simulink model "frontModel"  (R2020b)
settings: Solver=VariableStepAuto  StartTime=0.0  StopTime=10.0  RelTol=1e-3
model workspace: external: MATLAB File C:\Code\KillerWhaleSim\KillerWhaleSim\FrontParams.m (data not in the file)
undefined symbols (not defined in the file or in its folder): frontParams, X, Y, Z
libraries: sm_lib x1214, nesl_utility x1
(part 1 of 19)
settings Model: Creator=roadrunner  LastModifiedBy=roadrunner

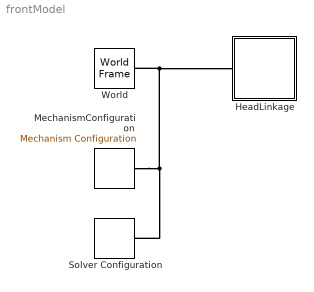
== system frontModel ==
  HeadLinkage : Subsystem
  MechanismConfiguration : sm_lib/Utilities/Mechanism Configuration  UniformGravity=Constant  GravityVector=[0 -9.80665 0]  GravityVectorUnits=m/s^2  GravityUnits=m/s^2  LinearizationDelta=0.001  JointModeTransitionNonlinearIterations=2
  Solver Configuration : nesl_utility/Solver Configuration  PhysicalDomain=network_engine_domain  SubClassName=solver  LeftPortType=input  RightPortType=generic  Tones=[]  Harmonics=[]  SimulateNoise=off  Profile=off  UseLocalSampling=off  EnableSwitchedLinearOptims=on  FrequencyDomain=off  UseCCode=off  RelTol=0.001  AbsTol=1e-06  MinStep=1e-09  ToWorkspace=off  RevertToSquareIcSolve=off  NumHomotopyIterations=100  PhasorMode=off  PhasorModeNumHarmonics=1  DoDC=off  ResidualTolerance=1e-09  UseLocalSolver=off  LocalSolverChoice=NE_BACKWARD_EULER_ADVANCER  LocalSolverSampleTime=0.001  DoFixedCost=off  MaxNonlinIter=3  MaxModeIter=2  ComputeImpulses=off  ImpulseIterations=2  LinearAlgebra=auto  EquationFormulation=NE_TIME_EF  DelaysMemoryBudget=1024  AutomaticFiltering=on  FilteringTimeConstant=0.001  PartitionStorageMethod=AS_NEEDED  PartitionMemoryBudget=1024  PartitionMethod=ROBUST
  World : sm_lib/Frames and Transforms/World Frame
  connections:
  World/RConn1 -- MechanismConfiguration/RConn1 -- Solver Configuration/RConn1 -- HeadLinkage/LConn1

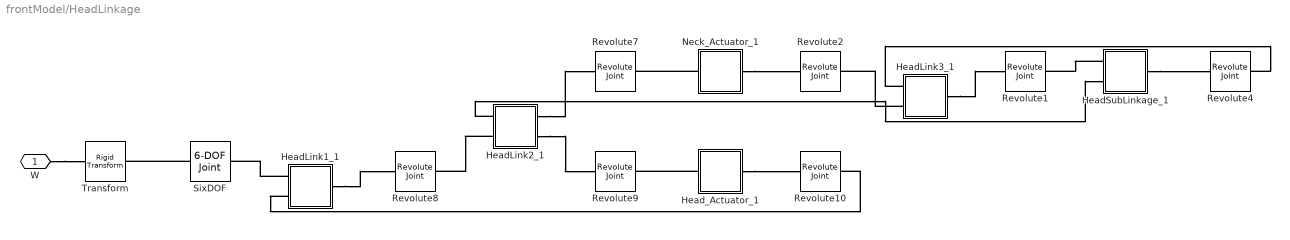
== system frontModel/HeadLinkage ==
  HeadLink1_1 : Subsystem
  HeadLink2_1 : Subsystem
  HeadLink3_1 : Subsystem
  HeadSubLinkage_1 : Subsystem
  Head_Actuator_1 : Subsystem
  Neck_Actuator_1 : Subsystem
  Revolute1 : sm_lib/Joints/Revolute Joint  JointMode=Normal  SenseConstraintForce=off  SenseConstraintForceX=off  SenseConstraintForceY=off  SenseConstraintForceZ=off  SenseConstraintTorque=off  SenseConstraintTorqueX=off  SenseConstraintTorqueY=off  SenseConstraintTorqueZ=off  SenseTotalForce=off  SenseTotalForceX=off  SenseTotalForceY=off  SenseTotalForceZ=off  SenseTotalTorque=off  SenseTotalTorqueX=off  SenseTotalTorqueY=off  SenseTotalTorqueZ=off  CompositeWrenchDir=FollowerOnBase  CompositeWrenchFrame=BaseFrame  EquilibriumPosition=0  EquilibriumPositionUnits=deg  SpringStiffness=0  SpringStiffnessUnits=N*m/deg  DampingCoefficient=0  DampingCoefficientUnits=N*m/(deg/s)  TorqueActuationMode=NoTorque  MotionActuationMode=ComputedMotion  SensePosition=off  SenseVelocity=off  SenseAcceleration=off  SenseTorqueForce=off  SenseLowerLimitTorqueForce=off  SenseUpperLimitTorqueForce=off  LowerLimitSpecify=off  LowerLimitBound=-90  LowerLimitBoundUnits=deg  LowerLimitStiffness=1e4  LowerLimitStiffnessUnits=N*m/deg  LowerLimitDamping=10  LowerLimitDampingUnits=N*m/(deg/s)  LowerLimitTransitionRegionWidth=0.1  LowerLimitTransitionRegionWidthUnits=deg  UpperLimitSpecify=off  UpperLimitBound=90  UpperLimitBoundUnits=deg  UpperLimitStiffness=1e4  UpperLimitStiffnessUnits=N*m/deg  UpperLimitDamping=10  UpperLimitDampingUnits=N*m/(deg/s)  UpperLimitTransitionRegionWidth=0.1  UpperLimitTransitionRegionWidthUnits=deg  PositionTargetSpecify=on  PositionTargetPriority=Low  PositionTargetValue=frontParams.RevoluteJoint(8).Rz.Pos  PositionTargetValueUnits=deg  VelocityTargetSpecify=off  VelocityTargetPriority=High  VelocityTargetValue=0  VelocityTargetValueUnits=deg/s
  Revolute10 : sm_lib/Joints/Revolute Joint  JointMode=Normal  SenseConstraintForce=off  SenseConstraintForceX=off  SenseConstraintForceY=off  SenseConstraintForceZ=off  SenseConstraintTorque=off  SenseConstraintTorqueX=off  SenseConstraintTorqueY=off  SenseConstraintTorqueZ=off  SenseTotalForce=off  SenseTotalForceX=off  SenseTotalForceY=off  SenseTotalForceZ=off  SenseTotalTorque=off  SenseTotalTorqueX=off  SenseTotalTorqueY=off  SenseTotalTorqueZ=off  CompositeWrenchDir=FollowerOnBase  CompositeWrenchFrame=BaseFrame  EquilibriumPosition=0  EquilibriumPositionUnits=deg  SpringStiffness=0  SpringStiffnessUnits=N*m/deg  DampingCoefficient=0  DampingCoefficientUnits=N*m/(deg/s)  TorqueActuationMode=NoTorque  MotionActuationMode=ComputedMotion  SensePosition=off  SenseVelocity=off  SenseAcceleration=off  SenseTorqueForce=off  SenseLowerLimitTorqueForce=off  SenseUpperLimitTorqueForce=off  LowerLimitSpecify=off  LowerLimitBound=-90  LowerLimitBoundUnits=deg  LowerLimitStiffness=1e4  LowerLimitStiffnessUnits=N*m/deg  LowerLimitDamping=10  LowerLimitDampingUnits=N*m/(deg/s)  LowerLimitTransitionRegionWidth=0.1  LowerLimitTransitionRegionWidthUnits=deg  UpperLimitSpecify=off  UpperLimitBound=90  UpperLimitBoundUnits=deg  UpperLimitStiffness=1e4  UpperLimitStiffnessUnits=N*m/deg  UpperLimitDamping=10  UpperLimitDampingUnits=N*m/(deg/s)  UpperLimitTransitionRegionWidth=0.1  UpperLimitTransitionRegionWidthUnits=deg  PositionTargetSpecify=on  PositionTargetPriority=Low  PositionTargetValue=frontParams.RevoluteJoint(5).Rz.Pos  PositionTargetValueUnits=deg  VelocityTargetSpecify=off  VelocityTargetPriority=High  VelocityTargetValue=0  VelocityTargetValueUnits=deg/s
  Revolute2 : sm_lib/Joints/Revolute Joint  JointMode=Normal  SenseConstraintForce=off  SenseConstraintForceX=off  SenseConstraintForceY=off  SenseConstraintForceZ=off  SenseConstraintTorque=off  SenseConstraintTorqueX=off  SenseConstraintTorqueY=off  SenseConstraintTorqueZ=off  SenseTotalForce=off  SenseTotalForceX=off  SenseTotalForceY=off  SenseTotalForceZ=off  SenseTotalTorque=off  SenseTotalTorqueX=off  SenseTotalTorqueY=off  SenseTotalTorqueZ=off  CompositeWrenchDir=FollowerOnBase  CompositeWrenchFrame=BaseFrame  EquilibriumPosition=0  EquilibriumPositionUnits=deg  SpringStiffness=0  SpringStiffnessUnits=N*m/deg  DampingCoefficient=0  DampingCoefficientUnits=N*m/(deg/s)  TorqueActuationMode=NoTorque  MotionActuationMode=ComputedMotion  SensePosition=off  SenseVelocity=off  SenseAcceleration=off  SenseTorqueForce=off  SenseLowerLimitTorqueForce=off  SenseUpperLimitTorqueForce=off  LowerLimitSpecify=off  LowerLimitBound=-90  LowerLimitBoundUnits=deg  LowerLimitStiffness=1e4  LowerLimitStiffnessUnits=N*m/deg  LowerLimitDamping=10  LowerLimitDampingUnits=N*m/(deg/s)  LowerLimitTransitionRegionWidth=0.1  LowerLimitTransitionRegionWidthUnits=deg  UpperLimitSpecify=off  UpperLimitBound=90  UpperLimitBoundUnits=deg  UpperLimitStiffness=1e4  UpperLimitStiffnessUnits=N*m/deg  UpperLimitDamping=10  UpperLimitDampingUnits=N*m/(deg/s)  UpperLimitTransitionRegionWidth=0.1  UpperLimitTransitionRegionWidthUnits=deg  PositionTargetSpecify=off  PositionTargetPriority=High  PositionTargetValue=0  PositionTargetValueUnits=deg  VelocityTargetSpecify=off  VelocityTargetPriority=High  VelocityTargetValue=0  VelocityTargetValueUnits=deg/s
  Revolute4 : sm_lib/Joints/Revolute Joint  JointMode=Normal  SenseConstraintForce=off  SenseConstraintForceX=off  SenseConstraintForceY=off  SenseConstraintForceZ=off  SenseConstraintTorque=off  SenseConstraintTorqueX=off  SenseConstraintTorqueY=off  SenseConstraintTorqueZ=off  SenseTotalForce=off  SenseTotalForceX=off  SenseTotalForceY=off  SenseTotalForceZ=off  SenseTotalTorque=off  SenseTotalTorqueX=off  SenseTotalTorqueY=off  SenseTotalTorqueZ=off  CompositeWrenchDir=FollowerOnBase  CompositeWrenchFrame=BaseFrame  EquilibriumPosition=0  EquilibriumPositionUnits=deg  SpringStiffness=0  SpringStiffnessUnits=N*m/deg  DampingCoefficient=0  DampingCoefficientUnits=N*m/(deg/s)  TorqueActuationMode=NoTorque  MotionActuationMode=ComputedMotion  SensePosition=off  SenseVelocity=off  SenseAcceleration=off  SenseTorqueForce=off  SenseLowerLimitTorqueForce=off  SenseUpperLimitTorqueForce=off  LowerLimitSpecify=off  LowerLimitBound=-90  LowerLimitBoundUnits=deg  LowerLimitStiffness=1e4  LowerLimitStiffnessUnits=N*m/deg  LowerLimitDamping=10  LowerLimitDampingUnits=N*m/(deg/s)  LowerLimitTransitionRegionWidth=0.1  LowerLimitTransitionRegionWidthUnits=deg  UpperLimitSpecify=off  UpperLimitBound=90  UpperLimitBoundUnits=deg  UpperLimitStiffness=1e4  UpperLimitStiffnessUnits=N*m/deg  UpperLimitDamping=10  UpperLimitDampingUnits=N*m/(deg/s)  UpperLimitTransitionRegionWidth=0.1  UpperLimitTransitionRegionWidthUnits=deg  PositionTargetSpecify=on  PositionTargetPriority=Low  PositionTargetValue=frontParams.RevoluteJoint(7).Rz.Pos  PositionTargetValueUnits=deg  VelocityTargetSpecify=off  VelocityTargetPriority=High  VelocityTargetValue=0  VelocityTargetValueUnits=deg/s
  Revolute7 : sm_lib/Joints/Revolute Joint  JointMode=Normal  SenseConstraintForce=off  SenseConstraintForceX=off  SenseConstraintForceY=off  SenseConstraintForceZ=off  SenseConstraintTorque=off  SenseConstraintTorqueX=off  SenseConstraintTorqueY=off  SenseConstraintTorqueZ=off  SenseTotalForce=off  SenseTotalForceX=off  SenseTotalForceY=off  SenseTotalForceZ=off  SenseTotalTorque=off  SenseTotalTorqueX=off  SenseTotalTorqueY=off  SenseTotalTorqueZ=off  CompositeWrenchDir=FollowerOnBase  CompositeWrenchFrame=BaseFrame  EquilibriumPosition=0  EquilibriumPositionUnits=deg  SpringStiffness=0  SpringStiffnessUnits=N*m/deg  DampingCoefficient=0  DampingCoefficientUnits=N*m/(deg/s)  TorqueActuationMode=NoTorque  MotionActuationMode=ComputedMotion  SensePosition=off  SenseVelocity=off  SenseAcceleration=off  SenseTorqueForce=off  SenseLowerLimitTorqueForce=off  SenseUpperLimitTorqueForce=off  LowerLimitSpecify=off  LowerLimitBound=-90  LowerLimitBoundUnits=deg  LowerLimitStiffness=1e4  LowerLimitStiffnessUnits=N*m/deg  LowerLimitDamping=10  LowerLimitDampingUnits=N*m/(deg/s)  LowerLimitTransitionRegionWidth=0.1  LowerLimitTransitionRegionWidthUnits=deg  UpperLimitSpecify=off  UpperLimitBound=90  UpperLimitBoundUnits=deg  UpperLimitStiffness=1e4  UpperLimitStiffnessUnits=N*m/deg  UpperLimitDamping=10  UpperLimitDampingUnits=N*m/(deg/s)  UpperLimitTransitionRegionWidth=0.1  UpperLimitTransitionRegionWidthUnits=deg  PositionTargetSpecify=on  PositionTargetPriority=Low  PositionTargetValue=frontParams.RevoluteJoint(9).Rz.Pos  PositionTargetValueUnits=deg  VelocityTargetSpecify=off  VelocityTargetPriority=High  VelocityTargetValue=0  VelocityTargetValueUnits=deg/s
  Revolute8 : sm_lib/Joints/Revolute Joint  JointMode=Normal  SenseConstraintForce=off  SenseConstraintForceX=off  SenseConstraintForceY=off  SenseConstraintForceZ=off  SenseConstraintTorque=off  SenseConstraintTorqueX=off  SenseConstraintTorqueY=off  SenseConstraintTorqueZ=off  SenseTotalForce=off  SenseTotalForceX=off  SenseTotalForceY=off  SenseTotalForceZ=off  SenseTotalTorque=off  SenseTotalTorqueX=off  SenseTotalTorqueY=off  SenseTotalTorqueZ=off  CompositeWrenchDir=FollowerOnBase  CompositeWrenchFrame=BaseFrame  EquilibriumPosition=0  EquilibriumPositionUnits=deg  SpringStiffness=0  SpringStiffnessUnits=N*m/deg  DampingCoefficient=0  DampingCoefficientUnits=N*m/(deg/s)  TorqueActuationMode=NoTorque  MotionActuationMode=ComputedMotion  SensePosition=off  SenseVelocity=off  SenseAcceleration=off  SenseTorqueForce=off  SenseLowerLimitTorqueForce=off  SenseUpperLimitTorqueForce=off  LowerLimitSpecify=off  LowerLimitBound=-90  LowerLimitBoundUnits=deg  LowerLimitStiffness=1e4  LowerLimitStiffnessUnits=N*m/deg  LowerLimitDamping=10  LowerLimitDampingUnits=N*m/(deg/s)  LowerLimitTransitionRegionWidth=0.1  LowerLimitTransitionRegionWidthUnits=deg  UpperLimitSpecify=off  UpperLimitBound=90  UpperLimitBoundUnits=deg  UpperLimitStiffness=1e4  UpperLimitStiffnessUnits=N*m/deg  UpperLimitDamping=10  UpperLimitDampingUnits=N*m/(deg/s)  UpperLimitTransitionRegionWidth=0.1  UpperLimitTransitionRegionWidthUnits=deg  PositionTargetSpecify=on  PositionTargetPriority=Low  PositionTargetValue=frontParams.RevoluteJoint(6).Rz.Pos  PositionTargetValueUnits=deg  VelocityTargetSpecify=off  VelocityTargetPriority=High  VelocityTargetValue=0  VelocityTargetValueUnits=deg/s
  Revolute9 : sm_lib/Joints/Revolute Joint  JointMode=Normal  SenseConstraintForce=off  SenseConstraintForceX=off  SenseConstraintForceY=off  SenseConstraintForceZ=off  SenseConstraintTorque=off  SenseConstraintTorqueX=off  SenseConstraintTorqueY=off  SenseConstraintTorqueZ=off  SenseTotalForce=off  SenseTotalForceX=off  SenseTotalForceY=off  SenseTotalForceZ=off  SenseTotalTorque=off  SenseTotalTorqueX=off  SenseTotalTorqueY=off  SenseTotalTorqueZ=off  CompositeWrenchDir=FollowerOnBase  CompositeWrenchFrame=BaseFrame  EquilibriumPosition=0  EquilibriumPositionUnits=deg  SpringStiffness=0  SpringStiffnessUnits=N*m/deg  DampingCoefficient=0  DampingCoefficientUnits=N*m/(deg/s)  TorqueActuationMode=NoTorque  MotionActuationMode=ComputedMotion  SensePosition=off  SenseVelocity=off  SenseAcceleration=off  SenseTorqueForce=off  SenseLowerLimitTorqueForce=off  SenseUpperLimitTorqueForce=off  LowerLimitSpecify=off  LowerLimitBound=-90  LowerLimitBoundUnits=deg  LowerLimitStiffness=1e4  LowerLimitStiffnessUnits=N*m/deg  LowerLimitDamping=10  LowerLimitDampingUnits=N*m/(deg/s)  LowerLimitTransitionRegionWidth=0.1  LowerLimitTransitionRegionWidthUnits=deg  UpperLimitSpecify=off  UpperLimitBound=90  UpperLimitBoundUnits=deg  UpperLimitStiffness=1e4  UpperLimitStiffnessUnits=N*m/deg  UpperLimitDamping=10  UpperLimitDampingUnits=N*m/(deg/s)  UpperLimitTransitionRegionWidth=0.1  UpperLimitTransitionRegionWidthUnits=deg  PositionTargetSpecify=off  PositionTargetPriority=High  PositionTargetValue=0  PositionTargetValueUnits=deg  VelocityTargetSpecify=off  VelocityTargetPriority=High  VelocityTargetValue=0  VelocityTargetValueUnits=deg/s
  SixDOF : sm_lib/Joints/6-DOF Joint  JointMode=Normal  SenseConstraintForce=off  SenseConstraintForceX=off  SenseConstraintForceY=off  SenseConstraintForceZ=off  SenseConstraintTorque=off  SenseConstraintTorqueX=off  SenseConstraintTorqueY=off  SenseConstraintTorqueZ=off  SenseTotalForce=off  SenseTotalForceX=off  SenseTotalForceY=off  SenseTotalForceZ=off  SenseTotalTorque=off  SenseTotalTorqueX=off  SenseTotalTorqueY=off  SenseTotalTorqueZ=off  CompositeWrenchDir=FollowerOnBase  CompositeWrenchFrame=BaseFrame  PxEquilibriumPosition=0  PxEquilibriumPositionUnits=m  PxSpringStiffness=0  PxSpringStiffnessUnits=N/m  PxDampingCoefficient=0  PxDampingCoefficientUnits=N/(m/s)  PxTorqueActuationMode=NoTorque  PxMotionActuationMode=ComputedMotion  PxSensePosition=off  PxSenseVelocity=off  PxSenseAcceleration=off  PxSenseTorqueForce=off  PxSenseLowerLimitTorqueForce=off  PxSenseUpperLimitTorqueForce=off  PxLowerLimitSpecify=off  PxLowerLimitBound=-1  PxLowerLimitBoundUnits=m  PxLowerLimitStiffness=1e6  PxLowerLimitStiffnessUnits=N/m  PxLowerLimitDamping=1e3  PxLowerLimitDampingUnits=N/(m/s)  PxLowerLimitTransitionRegionWidth=1e-4  PxLowerLimitTransitionRegionWidthUnits=m  PxUpperLimitSpecify=off  PxUpperLimitBound=1  PxUpperLimitBoundUnits=m  PxUpperLimitStiffness=1e6  PxUpperLimitStiffnessUnits=N/m  PxUpperLimitDamping=1e3  PxUpperLimitDampingUnits=N/(m/s)  PxUpperLimitTransitionRegionWidth=1e-4  PxUpperLimitTransitionRegionWidthUnits=m  PxPositionTargetSpecify=off  PxPositionTargetPriority=High  PxPositionTargetValue=0  PxPositionTargetValueUnits=m  PxVelocityTargetSpecify=off  PxVelocityTargetPriority=High  PxVelocityTargetValue=0  PxVelocityTargetValueUnits=m/s  PyEquilibriumPosition=0  PyEquilibriumPositionUnits=m  PySpringStiffness=0  PySpringStiffnessUnits=N/m  PyDampingCoefficient=0  PyDampingCoefficientUnits=N/(m/s)  PyTorqueActuationMode=NoTorque  PyMotionActuationMode=ComputedMotion  PySensePosition=off  PySenseVelocity=off  PySenseAcceleration=off  PySenseTorqueForce=off  PySenseLowerLimitTorqueForce=off  PySenseUpperLimitTorqueForce=off  PyLowerLimitSpecify=off  PyLowerLimitBound=-1  PyLowerLimitBoundUnits=m  PyLowerLimitStiffness=1e6  PyLowerLimitStiffnessUnits=N/m  PyLowerLimitDamping=1e3  PyLowerLimitDampingUnits=N/(m/s)  PyLowerLimitTransitionRegionWidth=1e-4  PyLowerLimitTransitionRegionWidthUnits=m  PyUpperLimitSpecify=off  PyUpperLimitBound=1  PyUpperLimitBoundUnits=m  PyUpperLimitStiffness=1e6  PyUpperLimitStiffnessUnits=N/m  PyUpperLimitDamping=1e3  PyUpperLimitDampingUnits=N/(m/s)  PyUpperLimitTransitionRegionWidth=1e-4  PyUpperLimitTransitionRegionWidthUnits=m  PyPositionTargetSpecify=off  PyPositionTargetPriority=High  PyPositionTargetValue=0  PyPositionTargetValueUnits=m  PyVelocityTargetSpecify=off  PyVelocityTargetPriority=High  PyVelocityTargetValue=0  PyVelocityTargetValueUnits=m/s  PzEquilibriumPosition=0  PzEquilibriumPositionUnits=m  PzSpringStiffness=0  PzSpringStiffnessUnits=N/m  PzDampingCoefficient=0  PzDampingCoefficientUnits=N/(m/s)  PzTorqueActuationMode=NoTorque  PzMotionActuationMode=ComputedMotion  PzSensePosition=off  PzSenseVelocity=off  PzSenseAcceleration=off  PzSenseTorqueForce=off  PzSenseLowerLimitTorqueForce=off  PzSenseUpperLimitTorqueForce=off  PzLowerLimitSpecify=off  PzLowerLimitBound=-1  PzLowerLimitBoundUnits=m  PzLowerLimitStiffness=1e6  PzLowerLimitStiffnessUnits=N/m  PzLowerLimitDamping=1e3  PzLowerLimitDampingUnits=N/(m/s)  PzLowerLimitTransitionRegionWidth=1e-4  PzLowerLimitTransitionRegionWidthUnits=m  PzUpperLimitSpecify=off  PzUpperLimitBound=1  PzUpperLimitBoundUnits=m  PzUpperLimitStiffness=1e6  PzUpperLimitStiffnessUnits=N/m  PzUpperLimitDamping=1e3  PzUpperLimitDampingUnits=N/(m/s)  PzUpperLimitTransitionRegionWidth=1e-4  PzUpperLimitTransitionRegionWidthUnits=m  PzPositionTargetSpecify=off  PzPositionTargetPriority=High  PzPositionTargetValue=0  PzPositionTargetValueUnits=m  PzVelocityTargetSpecify=off  PzVelocityTargetPriority=High  PzVelocityTargetValue=0  PzVelocityTargetValueUnits=m/s  SphDefPosRotationMethod=None  SphDefPosRotationAngleUnits=deg  SphDefPosRotationStandardAxis=+Z  SphDefPosRotationAngle=0.0  SphDefPosRotationArbitraryAxis=[0 0 1]  SphDefPosFollAlignAxisA=+X  SphDefPosBaseAlignAxisA=+Y  SphDefPosFollAlignAxisB=+Y  SphDefPosBaseAlignAxisB=+Z  SphDefPosRotationSequenceAxes=FollowerAxes  SphDefPosRotationSequence=XYX  SphDefPosRotationSequenceAngles=[0 0 0]  SphDefPosRotationSequenceAnglesUnits=deg  SphDefPosRotationMatrix=[1 0 0; 0 1 0; 0 0 1]  SphEqPosRotationMethod=None  SphEqPosRotationAngleUnits=deg  SphEqPosRotationStandardAxis=+Z  SphEqPosRotationAngle=0.0  SphEqPosRotationArbitraryAxis=[0 0 1]  SphEqPosFollAlignAxisA=+X  SphEqPosBaseAlignAxisA=+Y  SphEqPosFollAlignAxisB=+Y  SphEqPosBaseAlignAxisB=+Z  SphEqPosRotationSequenceAxes=FollowerAxes  SphEqPosRotationSequence=XYX  SphEqPosRotationSequenceAngles=[0 0 0]  SphEqPosRotationSequenceAnglesUnits=deg  SphEqPosRotationMatrix=[1 0 0; 0 1 0; 0 0 1]  SphSpringStiffness=0  SphSpringStiffnessUnits=N*m/deg  SphDampingCoefficient=0  SphDampingCoefficientUnits=N*m/(deg/s)  SphActuateTorqueX=off  SphActuateTorqueY=off  SphActuateTorqueZ=off  SphActuateTorque=off  SphTorqueActuationMode=NoTorque  SphMotionActuationMode=ComputedMotion  SphActuationFrame=BaseFrame  SphSensePosition=off  SphSenseVelocityX=off  SphSenseVelocityY=off  SphSenseVelocityZ=off  SphSenseVelocity=off  SphSenseAccelerationX=off  SphSenseAccelerationY=off  SphSenseAccelerationZ=off  SphSenseAcceleration=off  SphSenseTorqueX=off  SphSenseTorqueY=off  SphSenseTorqueZ=off  SphSenseTorqueForce=off  SphSenseLowerLimitTorqueMag=off  SphSenseUpperLimitTorqueMag=off  SphSensingFrame=FollowerFrame  SphLowerLimitSpecify=off  SphLowerLimitBound=15  SphLowerLimitBoundUnits=deg  SphLowerLimitStiffness=1e4  SphLowerLimitStiffnessUnits=N*m/deg  SphLowerLimitDamping=10  SphLowerLimitDampingUnits=N*m/(deg/s)  SphLowerLimitTransitionRegionWidth=0.1  SphLowerLimitTransitionRegionWidthUnits=deg  SphUpperLimitSpecify=off  SphUpperLimitBound=45  SphUpperLimitBoundUnits=deg  SphUpperLimitStiffness=1e4  SphUpperLimitStiffnessUnits=N*m/deg  SphUpperLimitDamping=10  SphUpperLimitDampingUnits=N*m/(deg/s)  SphUpperLimitTransitionRegionWidth=0.1  SphUpperLimitTransitionRegionWidthUnits=deg  SphPositionTargetRotationMethod=None  SphPositionTargetRotationAngleUnits=deg  SphPositionTargetRotationStandardAxis=+Z  SphPositionTargetRotationAngle=0.0  SphPositionTargetRotationArbitraryAxis=[0 0 1]  SphPositionTargetFollAlignAxisA=+X  SphPositionTargetBaseAlignAxisA=+Y  SphPositionTargetFollAlignAxisB=+Y  SphPositionTargetBaseAlignAxisB=+Z  SphPositionTargetRotationSequenceAxes=FollowerAxes  SphPositionTargetRotationSequence=XYX  SphPositionTargetRotationSequenceAngles=[0 0 0]  SphPositionTargetRotationSequenceAnglesUnits=deg  SphPositionTargetRotationMatrix=[1 0 0; 0 1 0; 0 0 1]  SphPositionTargetSpecify=off  SphPositionTargetPriority=High  SphVelocityTargetValue=[0 0 0]  SphVelocityTargetValueUnits=deg/s  SphVelocityTargetSpecify=off  SphVelocityTargetPriority=High  SphVelocityTargetInFollowerFrame=on
  Transform : sm_lib/Frames and Transforms/Rigid Transform  TranslationMethod=Cartesian  TranslationStandardOffset=0  TranslationLengthUnit=in  TranslationStandardAxis=+Z  TranslationCartesianOffset=frontParams.RigidTransform(423).translation  TranslationROffset=0  TranslationROffsetUnits=m  TranslationZOffset=0  TranslationZOffsetUnits=m  TranslationThetaOffset=0  TranslationThetaOffsetUnits=deg  RotationMethod=ArbitraryAxis  RotationAngleUnits=rad  RotationStandardAxis=+Z  RotationAngle=frontParams.RigidTransform(423).angle  RotationArbitraryAxis=frontParams.RigidTransform(423).axis  FollAlignAxisA=+X  BaseAlignAxisA=+Y  FollAlignAxisB=+Y  BaseAlignAxisB=+Z  RotationSequenceAxes=FollowerAxes  RotationSequence=XYX  RotationSequenceAngles=[0 0 0]  RotationSequenceAnglesUnits=deg  RotationMatrix=[1 0 0; 0 1 0; 0 0 1]
  W : PMIOPort  Side=Left
  connections:
  HeadSubLinkage_1/LConn1 -- Revolute1/RConn1
  HeadLink2_1/RConn2 -- Revolute9/LConn1
  Head_Actuator_1/RConn1 -- Revolute10/LConn1
  Neck_Actuator_1/LConn1 -- Revolute7/RConn1
  HeadLink2_1/LConn2 -- Revolute8/RConn1
  HeadLink1_1/RConn1 -- Revolute8/LConn1
  HeadLink3_1/LConn1 -- Revolute4/RConn1
  HeadLink1_1/LConn1 -- SixDOF/RConn1
  SixDOF/LConn1 -- Transform/RConn1
  HeadLink1_1/LConn2 -- Revolute10/RConn1
  HeadSubLinkage_1/RConn1 -- Revolute4/LConn1
  HeadLink2_1/LConn1 -- HeadSubLinkage_1/LConn2
  Head_Actuator_1/LConn1 -- Revolute9/RConn1
  Neck_Actuator_1/RConn1 -- Revolute2/LConn1
  HeadLink3_1/RConn1 -- Revolute1/LConn1
  HeadLink3_1/LConn2 -- Revolute2/RConn1
  HeadLink2_1/RConn1 -- Revolute7/LConn1
  W/RConn1 -- Transform/LConn1

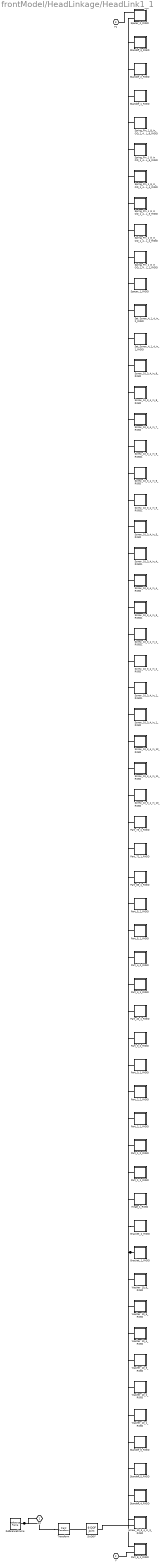
== system frontModel/HeadLinkage/HeadLink1_1 ==
  Bracket_1_RIGID : Subsystem
  Bracket_2_RIGID : Subsystem
  Hinge_1_RIGID : Subsystem
  Part_1_1_RIGID : Subsystem
  Part_1_2_RIGID : Subsystem
  Part_2_1_RIGID : Subsystem
  Part_2_2_RIGID : Subsystem
  Part_3_1_RIGID : Subsystem
  Part_3_2_RIGID : Subsystem
  Part_40_1_RIGID : Subsystem
  Part_4_1_RIGID : Subsystem
  Part_4_2_RIGID : Subsystem
  Part_5_1_RIGID : Subsystem
  Part_5_2_RIGID : Subsystem
  Part_65_1_RIGID : Subsystem
  Part_6_1_RIGID : Subsystem
  Part_72_1_RIGID : Subsystem
  Part_73_1_RIGID : Subsystem
  ReferenceFrame : sm_lib/Frames and Transforms/Reference Frame
  Screw_10_3_4_in_10_RIGID : Subsystem
  Screw_10_3_4_in_11_RIGID : Subsystem
  Screw_10_3_4_in_12_RIGID : Subsystem
  Screw_10_3_4_in_1_RIGID : Subsystem
  Screw_10_3_4_in_1_RIGID1 : Subsystem
  Screw_10_3_4_in_2_RIGID : Subsystem
  Screw_10_3_4_in_2_RIGID1 : Subsystem
  Screw_10_3_4_in_3_RIGID : Subsystem
  Screw_10_3_4_in_3_RIGID1 : Subsystem
  Screw_10_3_4_in_4_RIGID : Subsystem
  Screw_10_3_4_in_4_RIGID1 : Subsystem
  Screw_10_3_4_in_5_RIGID : Subsystem
  Screw_10_3_4_in_5_RIGID1 : Subsystem
  Screw_10_3_4_in_6_RIGID : Subsystem
  Screw_10_3_4_in_6_RIGID1 : Subsystem
  Screw_10_3_4_in_7_RIGID : Subsystem
  Screw_10_3_4_in_8_RIGID : Subsystem
  Screw_10_3_4_in_9_RIGID : Subsystem
  Set_Screw_4_1_4_in_1_RIGID : Subsystem
  Set_Screw_4_1_4_in_2_RIGID : Subsystem
  SixDOF : sm_lib/Joints/6-DOF Joint  JointMode=Normal  SenseConstraintForce=off  SenseConstraintForceX=off  SenseConstraintForceY=off  SenseConstraintForceZ=off  SenseConstraintTorque=off  SenseConstraintTorqueX=off  SenseConstraintTorqueY=off  SenseConstraintTorqueZ=off  SenseTotalForce=off  SenseTotalForceX=off  SenseTotalForceY=off  SenseTotalForceZ=off  SenseTotalTorque=off  SenseTotalTorqueX=off  SenseTotalTorqueY=off  SenseTotalTorqueZ=off  CompositeWrenchDir=FollowerOnBase  CompositeWrenchFrame=BaseFrame  PxEquilibriumPosition=0  PxEquilibriumPositionUnits=m  PxSpringStiffness=0  PxSpringStiffnessUnits=N/m  PxDampingCoefficient=0  PxDampingCoefficientUnits=N/(m/s)  PxTorqueActuationMode=NoTorque  PxMotionActuationMode=ComputedMotion  PxSensePosition=off  PxSenseVelocity=off  PxSenseAcceleration=off  PxSenseTorqueForce=off  PxSenseLowerLimitTorqueForce=off  PxSenseUpperLimitTorqueForce=off  PxLowerLimitSpecify=off  PxLowerLimitBound=-1  PxLowerLimitBoundUnits=m  PxLowerLimitStiffness=1e6  PxLowerLimitStiffnessUnits=N/m  PxLowerLimitDamping=1e3  PxLowerLimitDampingUnits=N/(m/s)  PxLowerLimitTransitionRegionWidth=1e-4  PxLowerLimitTransitionRegionWidthUnits=m  PxUpperLimitSpecify=off  PxUpperLimitBound=1  PxUpperLimitBoundUnits=m  PxUpperLimitStiffness=1e6  PxUpperLimitStiffnessUnits=N/m  PxUpperLimitDamping=1e3  PxUpperLimitDampingUnits=N/(m/s)  PxUpperLimitTransitionRegionWidth=1e-4  PxUpperLimitTransitionRegionWidthUnits=m  PxPositionTargetSpecify=off  PxPositionTargetPriority=High  PxPositionTargetValue=0  PxPositionTargetValueUnits=m  PxVelocityTargetSpecify=off  PxVelocityTargetPriority=High  PxVelocityTargetValue=0  PxVelocityTargetValueUnits=m/s  PyEquilibriumPosition=0  PyEquilibriumPositionUnits=m  PySpringStiffness=0  PySpringStiffnessUnits=N/m  PyDampingCoefficient=0  PyDampingCoefficientUnits=N/(m/s)  PyTorqueActuationMode=NoTorque  PyMotionActuationMode=ComputedMotion  PySensePosition=off  PySenseVelocity=off  PySenseAcceleration=off  PySenseTorqueForce=off  PySenseLowerLimitTorqueForce=off  PySenseUpperLimitTorqueForce=off  PyLowerLimitSpecify=off  PyLowerLimitBound=-1  PyLowerLimitBoundUnits=m  PyLowerLimitStiffness=1e6  PyLowerLimitStiffnessUnits=N/m  PyLowerLimitDamping=1e3  PyLowerLimitDampingUnits=N/(m/s)  PyLowerLimitTransitionRegionWidth=1e-4  PyLowerLimitTransitionRegionWidthUnits=m  PyUpperLimitSpecify=off  PyUpperLimitBound=1  PyUpperLimitBoundUnits=m  PyUpperLimitStiffness=1e6  PyUpperLimitStiffnessUnits=N/m  PyUpperLimitDamping=1e3  PyUpperLimitDampingUnits=N/(m/s)  PyUpperLimitTransitionRegionWidth=1e-4  PyUpperLimitTransitionRegionWidthUnits=m  PyPositionTargetSpecify=off  PyPositionTargetPriority=High  PyPositionTargetValue=0  PyPositionTargetValueUnits=m  PyVelocityTargetSpecify=off  PyVelocityTargetPriority=High  PyVelocityTargetValue=0  PyVelocityTargetValueUnits=m/s  PzEquilibriumPosition=0  PzEquilibriumPositionUnits=m  PzSpringStiffness=0  PzSpringStiffnessUnits=N/m  PzDampingCoefficient=0  PzDampingCoefficientUnits=N/(m/s)  PzTorqueActuationMode=NoTorque  PzMotionActuationMode=ComputedMotion  PzSensePosition=off  PzSenseVelocity=off  PzSenseAcceleration=off  PzSenseTorqueForce=off  PzSenseLowerLimitTorqueForce=off  PzSenseUpperLimitTorqueForce=off  PzLowerLimitSpecify=off  PzLowerLimitBound=-1  PzLowerLimitBoundUnits=m  PzLowerLimitStiffness=1e6  PzLowerLimitStiffnessUnits=N/m  PzLowerLimitDamping=1e3  PzLowerLimitDampingUnits=N/(m/s)  PzLowerLimitTransitionRegionWidth=1e-4  PzLowerLimitTransitionRegionWidthUnits=m  PzUpperLimitSpecify=off  PzUpperLimitBound=1  PzUpperLimitBoundUnits=m  PzUpperLimitStiffness=1e6  PzUpperLimitStiffnessUnits=N/m  PzUpperLimitDamping=1e3  PzUpperLimitDampingUnits=N/(m/s)  PzUpperLimitTransitionRegionWidth=1e-4  PzUpperLimitTransitionRegionWidthUnits=m  PzPositionTargetSpecify=off  PzPositionTargetPriority=High  PzPositionTargetValue=0  PzPositionTargetValueUnits=m  PzVelocityTargetSpecify=off  PzVelocityTargetPriority=High  PzVelocityTargetValue=0  PzVelocityTargetValueUnits=m/s  SphDefPosRotationMethod=None  SphDefPosRotationAngleUnits=deg  SphDefPosRotationStandardAxis=+Z  SphDefPosRotationAngle=0.0  SphDefPosRotationArbitraryAxis=[0 0 1]  SphDefPosFollAlignAxisA=+X  SphDefPosBaseAlignAxisA=+Y  SphDefPosFollAlignAxisB=+Y  SphDefPosBaseAlignAxisB=+Z  SphDefPosRotationSequenceAxes=FollowerAxes  SphDefPosRotationSequence=XYX  SphDefPosRotationSequenceAngles=[0 0 0]  SphDefPosRotationSequenceAnglesUnits=deg  SphDefPosRotationMatrix=[1 0 0; 0 1 0; 0 0 1]  SphEqPosRotationMethod=None  SphEqPosRotationAngleUnits=deg  SphEqPosRotationStandardAxis=+Z  SphEqPosRotationAngle=0.0  SphEqPosRotationArbitraryAxis=[0 0 1]  SphEqPosFollAlignAxisA=+X  SphEqPosBaseAlignAxisA=+Y  SphEqPosFollAlignAxisB=+Y  SphEqPosBaseAlignAxisB=+Z  SphEqPosRotationSequenceAxes=FollowerAxes  SphEqPosRotationSequence=XYX  SphEqPosRotationSequenceAngles=[0 0 0]  SphEqPosRotationSequenceAnglesUnits=deg  SphEqPosRotationMatrix=[1 0 0; 0 1 0; 0 0 1]  SphSpringStiffness=0  SphSpringStiffnessUnits=N*m/deg  SphDampingCoefficient=0  SphDampingCoefficientUnits=N*m/(deg/s)  SphActuateTorqueX=off  SphActuateTorqueY=off  SphActuateTorqueZ=off  SphActuateTorque=off  SphTorqueActuationMode=NoTorque  SphMotionActuationMode=ComputedMotion  SphActuationFrame=BaseFrame  SphSensePosition=off  SphSenseVelocityX=off  SphSenseVelocityY=off  SphSenseVelocityZ=off  SphSenseVelocity=off  SphSenseAccelerationX=off  SphSenseAccelerationY=off  SphSenseAccelerationZ=off  SphSenseAcceleration=off  SphSenseTorqueX=off  SphSenseTorqueY=off  SphSenseTorqueZ=off  SphSenseTorqueForce=off  SphSenseLowerLimitTorqueMag=off  SphSenseUpperLimitTorqueMag=off  SphSensingFrame=FollowerFrame  SphLowerLimitSpecify=off  SphLowerLimitBound=15  SphLowerLimitBoundUnits=deg  SphLowerLimitStiffness=1e4  SphLowerLimitStiffnessUnits=N*m/deg  SphLowerLimitDamping=10  SphLowerLimitDampingUnits=N*m/(deg/s)  SphLowerLimitTransitionRegionWidth=0.1  SphLowerLimitTransitionRegionWidthUnits=deg  SphUpperLimitSpecify=off  SphUpperLimitBound=45  SphUpperLimitBoundUnits=deg  SphUpperLimitStiffness=1e4  SphUpperLimitStiffnessUnits=N*m/deg  SphUpperLimitDamping=10  SphUpperLimitDampingUnits=N*m/(deg/s)  SphUpperLimitTransitionRegionWidth=0.1  SphUpperLimitTransitionRegionWidthUnits=deg  SphPositionTargetRotationMethod=None  SphPositionTargetRotationAngleUnits=deg  SphPositionTargetRotationStandardAxis=+Z  SphPositionTargetRotationAngle=0.0  SphPositionTargetRotationArbitraryAxis=[0 0 1]  SphPositionTargetFollAlignAxisA=+X  SphPositionTargetBaseAlignAxisA=+Y  SphPositionTargetFollAlignAxisB=+Y  SphPositionTargetBaseAlignAxisB=+Z  SphPositionTargetRotationSequenceAxes=FollowerAxes  SphPositionTargetRotationSequence=XYX  SphPositionTargetRotationSequenceAngles=[0 0 0]  SphPositionTargetRotationSequenceAnglesUnits=deg  SphPositionTargetRotationMatrix=[1 0 0; 0 1 0; 0 0 1]  SphPositionTargetSpecify=off  SphPositionTargetPriority=High  SphVelocityTargetValue=[0 0 0]  SphVelocityTargetValueUnits=deg/s  SphVelocityTargetSpecify=off  SphVelocityTargetPriority=High  SphVelocityTargetInFollowerFrame=on
  Spacer_1_RIGID : Subsystem
  Spacer_2_RIGID : Subsystem
  Spring_Pin_1_8_in_OD_1_4_in_L_1_RIGID : Subsystem
  Spring_Pin_1_8_in_OD_1_4_in_L_2_RIGID : Subsystem
  Spring_Pin_1_8_in_OD_1_4_in_L_3_RIGID : Subsystem
  Spring_Pin_1_8_in_OD_1_4_in_L_4_RIGID : Subsystem
  Spring_Pin_1_8_in_OD_1_4_in_L_5_RIGID : Subsystem
  Spring_Pin_1_8_in_OD_1_4_in_L_6_RIGID : Subsystem
  Standoff_1_RIGID : Subsystem
  Standoff_2_RIGID : Subsystem
  Standoff_3_RIGID : Subsystem
  Standoff_4_RIGID : Subsystem
  Standoff_5_RIGID : Subsystem
  Standoff_6_RIGID : Subsystem
  Transform : sm_lib/Frames and Transforms/Rigid Transform  TranslationMethod=Cartesian  TranslationStandardOffset=0  TranslationLengthUnit=in  TranslationStandardAxis=+Z  TranslationCartesianOffset=frontParams.RigidTransform(424).translation  TranslationROffset=0  TranslationROffsetUnits=m  TranslationZOffset=0  TranslationZOffsetUnits=m  TranslationThetaOffset=0  TranslationThetaOffsetUnits=deg  RotationMethod=ArbitraryAxis  RotationAngleUnits=rad  RotationStandardAxis=+Z  RotationAngle=frontParams.RigidTransform(424).angle  RotationArbitraryAxis=frontParams.RigidTransform(424).axis  FollAlignAxisA=+X  BaseAlignAxisA=+Y  FollAlignAxisB=+Y  BaseAlignAxisB=+Z  RotationSequenceAxes=FollowerAxes  RotationSequence=XYX  RotationSequenceAngles=[0 0 0]  RotationSequenceAnglesUnits=deg  RotationMatrix=[1 0 0; 0 1 0; 0 0 1]
  Washer_10_1_RIGID : Subsystem
  Washer_10_2_RIGID : Subsystem
  Washer_10_3_RIGID : Subsystem
  Washer_10_4_RIGID : Subsystem
  Washer_10_5_RIGID : Subsystem
  Washer_10_6_RIGID : Subsystem
  F2 : PMIOPort  Side=Left
  F : PMIOPort  Port=2  Side=Left
  F1 : PMIOPort  Port=3  Side=Right
  connections:
  Bracket_2_RIGID/LConn1 -- Bracket_1_RIGID/LConn1 -- Hinge_1_RIGID/LConn1 -- Part_1_1_RIGID/LConn1 -- Part_1_2_RIGID/LConn1 -- Part_2_1_RIGID/LConn1 -- Part_2_2_RIGID/LConn1 -- Part_3_1_RIGID/LConn1 -- Part_3_2_RIGID/LConn1 -- Part_40_1_RIGID/LConn1 -- Part_4_1_RIGID/LConn1 -- Part_4_2_RIGID/LConn1 -- Part_5_1_RIGID/LConn1 -- Part_5_2_RIGID/LConn1 -- Part_65_1_RIGID/LConn1 -- Part_6_1_RIGID/LConn1 -- Part_72_1_RIGID/LConn1 -- Part_73_1_RIGID/LConn1 -- Screw_10_3_4_in_10_RIGID/LConn1 -- Screw_10_3_4_in_11_RIGID/LConn1 -- Screw_10_3_4_in_12_RIGID/LConn1 -- Screw_10_3_4_in_1_RIGID/LConn1 -- Screw_10_3_4_in_1_RIGID1/LConn1 -- Screw_10_3_4_in_2_RIGID/LConn1 -- Screw_10_3_4_in_2_RIGID1/LConn1 -- Screw_10_3_4_in_3_RIGID/LConn1 -- Screw_10_3_4_in_3_RIGID1/LConn1 -- Screw_10_3_4_in_4_RIGID/LConn1 -- Screw_10_3_4_in_4_RIGID1/LConn1 -- Screw_10_3_4_in_5_RIGID/LConn1 -- Screw_10_3_4_in_5_RIGID1/LConn1 -- Screw_10_3_4_in_6_RIGID/LConn1 -- Screw_10_3_4_in_6_RIGID1/LConn1 -- Screw_10_3_4_in_7_RIGID/LConn1 -- Screw_10_3_4_in_8_RIGID/LConn1 -- Screw_10_3_4_in_9_RIGID/LConn1 -- Set_Screw_4_1_4_in_1_RIGID/LConn1 -- Set_Screw_4_1_4_in_2_RIGID/LConn1 -- Spacer_1_RIGID/LConn1 -- Spacer_2_RIGID/LConn2 -- Spring_Pin_1_8_in_OD_1_4_in_L_1_RIGID/LConn1 -- Spring_Pin_1_8_in_OD_1_4_in_L_2_RIGID/LConn1 -- Spring_Pin_1_8_in_OD_1_4_in_L_3_RIGID/LConn1 -- Spring_Pin_1_8_in_OD_1_4_in_L_4_RIGID/LConn1 -- Spring_Pin_1_8_in_OD_1_4_in_L_5_RIGID/LConn1 -- Spring_Pin_1_8_in_OD_1_4_in_L_6_RIGID/LConn1 -- Standoff_1_RIGID/LConn1 -- Standoff_2_RIGID/LConn1 -- Standoff_3_RIGID/LConn1 -- Standoff_4_RIGID/LConn1 -- Standoff_5_RIGID/LConn1 -- Standoff_6_RIGID/LConn1 -- Washer_10_1_RIGID/LConn1 -- Washer_10_2_RIGID/LConn1 -- Washer_10_3_RIGID/LConn1 -- Washer_10_4_RIGID/LConn1 -- Washer_10_5_RIGID/LConn1 -- Washer_10_6_RIGID/LConn1
  Part_6_1_RIGID/LConn2 -- F/RConn1
  Spacer_2_RIGID/LConn1 -- F1/RConn1
  Transform/LConn1 -- ReferenceFrame/RConn1 -- F2/RConn1
  Screw_10_3_4_in_3_RIGID/LConn2 -- SixDOF/RConn1
  SixDOF/LConn1 -- Transform/RConn1

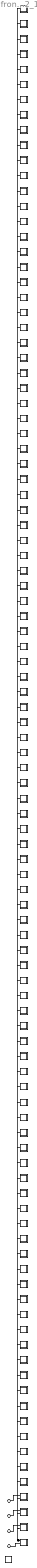
== system frontModel/HeadLinkage/HeadLink2_1 ==
  Frame_Part_1_RIGID : Subsystem
  Frame_Part_2_RIGID : Subsystem
  Part_1_1_RIGID : Subsystem
  Part_1_2_RIGID : Subsystem
  Part_1_3_RIGID : Subsystem
  Part_1_4_RIGID : Subsystem
  Part_24_1_RIGID : Subsystem
  Part_24r_1_RIGID : Subsystem
  Part_2_1_RIGID : Subsystem
  Part_2_2_RIGID : Subsystem
  Part_2_3_RIGID : Subsystem
  Part_2_4_RIGID : Subsystem
  Part_3_1_RIGID : Subsystem
  Part_3_2_RIGID : Subsystem
  Part_3_3_RIGID : Subsystem
  Part_3_4_RIGID : Subsystem
  Part_4_1_RIGID : Subsystem
  Part_4_2_RIGID : Subsystem
  Part_4_3_RIGID : Subsystem
  Part_4_4_RIGID : Subsystem
  Part_5_1_RIGID : Subsystem
  Part_5_2_RIGID : Subsystem
  Part_5_3_RIGID : Subsystem
  Part_5_4_RIGID : Subsystem
  Part_6_1_RIGID : Subsystem
  Part_6_2_RIGID : Subsystem
  Part_809_1_RIGID : Subsystem
  Part_809_2_RIGID : Subsystem
  Part_809_3_RIGID : Subsystem
  Part_809_4_RIGID : Subsystem
  Part_809_5_RIGID : Subsystem
  Part_811_1_RIGID : Subsystem
  Part_812_1_RIGID : Subsystem
  Part_813_1_RIGID : Subsystem
  Part_814_1_RIGID : Subsystem
  Part_815_1_RIGID : Subsystem
  Part_816_1_RIGID : Subsystem
  Part_817_1_RIGID : Subsystem
  Part_818_1_RIGID : Subsystem
  Part_819_1_RIGID : Subsystem
  Part_820_1_RIGID : Subsystem
  Part_821_1_RIGID : Subsystem
  Part_822_1_RIGID : Subsystem
  Part_823_1_RIGID : Subsystem
  Part_824_1_RIGID : Subsystem
  Part_824_2_RIGID : Subsystem
  Part_825_1_RIGID : Subsystem
  Part_825_2_RIGID : Subsystem
  Part_826_1_RIGID : Subsystem
  Part_826_2_RIGID : Subsystem
  Part_827_1_RIGID : Subsystem
  Part_827_2_RIGID : Subsystem
  Part_828_1_RIGID : Subsystem
  Part_828_2_RIGID : Subsystem
  Part_867_1_RIGID : Subsystem
  Part_870_1_RIGID : Subsystem
  Part_875_1_RIGID : Subsystem
  Part_936_1_RIGID : Subsystem
  Part_937_1_RIGID : Subsystem
  Part_938_1_RIGID : Subsystem
  Part_939_1_RIGID : Subsystem
  ReferenceFrame : sm_lib/Frames and Transforms/Reference Frame
  Screw_10_3_4_in_1_RIGID : Subsystem
  Screw_10_3_4_in_2_RIGID : Subsystem
  Screw_10_3_4_in_3_RIGID : Subsystem
  Screw_10_3_4_in_4_RIGID : Subsystem
  Screw_10_3_4_in_5_RIGID : Subsystem
  Screw_10_3_4_in_6_RIGID : Subsystem
  Screw_8_1_2_in_1_RIGID : Subsystem
  Screw_8_1_2_in_2_RIGID : Subsystem
  Spring_Pin_1_8_in_OD_1_4_in_L_1_RIGID : Subsystem
  Spring_Pin_1_8_in_OD_1_4_in_L_2_RIGID : Subsystem
  Spring_Pin_1_8_in_OD_1_4_in_L_3_RIGID : Subsystem
  Spring_Pin_1_8_in_OD_1_4_in_L_4_RIGID : Subsystem
  Spring_Pin_1_8_in_OD_1_4_in_L_5_RIGID : Subsystem
  Spring_Pin_1_8_in_OD_1_4_in_L_6_RIGID : Subsystem
  Standoff_1_RIGID : Subsystem
  Washer_10_10_RIGID : Subsystem
  Washer_10_1_RIGID : Subsystem
  Washer_10_2_RIGID : Subsystem
  Washer_10_3_RIGID : Subsystem
  Washer_10_4_RIGID : Subsystem
  Washer_10_5_RIGID : Subsystem
  Washer_10_6_RIGID : Subsystem
  Washer_10_7_RIGID : Subsystem
  Washer_10_8_RIGID : Subsystem
  Washer_10_9_RIGID : Subsystem
  Washer_8_1_RIGID : Subsystem
  Washer_8_2_RIGID : Subsystem
  bulkheads7_1_RIGID : Subsystem
  bulkheads7_2_RIGID : Subsystem
  bulkheads7_3_RIGID : Subsystem
  bulkheads7_4_RIGID : Subsystem
  bulkheads7_5_RIGID : Subsystem
  bulkheads8_1_RIGID : Subsystem
  bulkheads8_2_RIGID : Subsystem
  bulkheads8_3_RIGID : Subsystem
  bulkheads8_4_RIGID : Subsystem
  bulkheads8_5_RIGID : Subsystem
  nut_1_RIGID : Subsystem
  nut_2_RIGID : Subsystem
  nut_3_RIGID : Subsystem
  nut_4_RIGID : Subsystem
  F2 : PMIOPort  Side=Left
  F1 : PMIOPort  Port=2  Side=Left
  F4 : PMIOPort  Port=3  Side=Right
  F : PMIOPort  Port=4  Side=Right
  connections:
  Frame_Part_2_RIGID/LConn2 -- Frame_Part_1_RIGID/LConn1 -- Part_1_1_RIGID/LConn1 -- Part_1_2_RIGID/LConn1 -- Part_1_3_RIGID/LConn2 -- Part_1_4_RIGID/LConn2 -- Part_24_1_RIGID/LConn1 -- Part_24r_1_RIGID/LConn1 -- Part_2_1_RIGID/LConn1 -- Part_2_2_RIGID/LConn1 -- Part_2_3_RIGID/LConn1 -- Part_2_4_RIGID/LConn1 -- Part_3_1_RIGID/LConn1 -- Part_3_2_RIGID/LConn1 -- Part_3_3_RIGID/LConn1 -- Part_3_4_RIGID/LConn1 -- Part_4_1_RIGID/LConn1 -- Part_4_2_RIGID/LConn1 -- Part_4_3_RIGID/LConn1 -- Part_4_4_RIGID/LConn1 -- Part_5_1_RIGID/LConn1 -- Part_5_2_RIGID/LConn1 -- Part_5_3_RIGID/LConn1 -- Part_5_4_RIGID/LConn1 -- Part_6_1_RIGID/LConn1 -- Part_6_2_RIGID/LConn1 -- Part_809_1_RIGID/LConn1 -- Part_809_2_RIGID/LConn1 -- Part_809_3_RIGID/LConn1 -- Part_809_4_RIGID/LConn1 -- Part_809_5_RIGID/LConn1 -- Part_811_1_RIGID/LConn1 -- Part_812_1_RIGID/LConn1 -- Part_813_1_RIGID/LConn1 -- Part_814_1_RIGID/LConn1 -- Part_815_1_RIGID/LConn1 -- Part_816_1_RIGID/LConn1 -- Part_817_1_RIGID/LConn1 -- Part_818_1_RIGID/LConn1 -- Part_819_1_RIGID/LConn1 -- Part_820_1_RIGID/LConn1 -- Part_821_1_RIGID/LConn1 -- Part_822_1_RIGID/LConn1 -- Part_823_1_RIGID/LConn1 -- Part_824_1_RIGID/LConn1 -- Part_824_2_RIGID/LConn1 -- Part_825_1_RIGID/LConn1 -- Part_825_2_RIGID/LConn1 -- Part_826_1_RIGID/LConn1 -- Part_826_2_RIGID/LConn1 -- Part_827_1_RIGID/LConn1 -- Part_827_2_RIGID/LConn1 -- Part_828_1_RIGID/LConn1 -- Part_828_2_RIGID/LConn1 -- Part_867_1_RIGID/LConn1 -- Part_870_1_RIGID/LConn1 -- Part_875_1_RIGID/LConn1 -- Part_936_1_RIGID/LConn1 -- Part_937_1_RIGID/LConn1 -- Part_938_1_RIGID/LConn1 -- Part_939_1_RIGID/LConn1 -- Screw_10_3_4_in_1_RIGID/LConn1 -- Screw_10_3_4_in_2_RIGID/LConn1 -- Screw_10_3_4_in_3_RIGID/LConn1 -- Screw_10_3_4_in_4_RIGID/LConn1 -- Screw_10_3_4_in_5_RIGID/LConn1 -- Screw_10_3_4_in_6_RIGID/LConn1 -- Screw_8_1_2_in_1_RIGID/LConn1 -- Screw_8_1_2_in_2_RIGID/LConn1 -- Spring_Pin_1_8_in_OD_1_4_in_L_1_RIGID/LConn1 -- Spring_Pin_1_8_in_OD_1_4_in_L_2_RIGID/LConn1 -- Spring_Pin_1_8_in_OD_1_4_in_L_3_RIGID/LConn1 -- Spring_Pin_1_8_in_OD_1_4_in_L_4_RIGID/LConn1 -- Spring_Pin_1_8_in_OD_1_4_in_L_5_RIGID/LConn1 -- Spring_Pin_1_8_in_OD_1_4_in_L_6_RIGID/LConn1 -- Standoff_1_RIGID/LConn1 -- Washer_10_10_RIGID/LConn1 -- Washer_10_1_RIGID/LConn1 -- Washer_10_2_RIGID/LConn1 -- Washer_10_3_RIGID/LConn1 -- Washer_10_4_RIGID/LConn1 -- Washer_10_5_RIGID/LConn1 -- Washer_10_6_RIGID/LConn1 -- Washer_10_7_RIGID/LConn1 -- Washer_10_8_RIGID/LConn1 -- Washer_10_9_RIGID/LConn1 -- Washer_8_1_RIGID/LConn1 -- Washer_8_2_RIGID/LConn1 -- bulkheads7_1_RIGID/LConn1 -- bulkheads7_2_RIGID/LConn1 -- bulkheads7_3_RIGID/LConn1 -- bulkheads7_4_RIGID/LConn1 -- bulkheads7_5_RIGID/LConn1 -- bulkheads8_1_RIGID/LConn1 -- bulkheads8_2_RIGID/LConn1 -- bulkheads8_3_RIGID/LConn1 -- bulkheads8_4_RIGID/LConn1 -- bulkheads8_5_RIGID/LConn1 -- nut_1_RIGID/LConn1 -- nut_2_RIGID/LConn1 -- nut_3_RIGID/LConn1 -- nut_4_RIGID/LConn1
  Part_1_4_RIGID/LConn1 -- F/RConn1
  Frame_Part_1_RIGID/LConn2 -- F1/RConn1
  Frame_Part_2_RIGID/LConn1 -- F2/RConn1
  Part_1_3_RIGID/LConn1 -- F4/RConn1

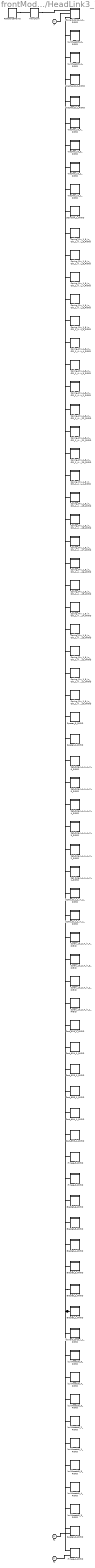
== system frontModel/HeadLinkage/HeadLink3_1 ==
  Bracket_1_RIGID : Subsystem
  Bracket_2_RIGID : Subsystem
  Bracket_3_RIGID : Subsystem
  Bracket_4_RIGID : Subsystem
  Bracket_5_RIGID : Subsystem
  Bracket_6_RIGID : Subsystem
  Hinge_1_RIGID : Subsystem
  Hinge_2_RIGID : Subsystem
  Hinge_3_RIGID : Subsystem
  Part_853_1_RIGID : Subsystem
  Part_854_1_RIGID : Subsystem
  Part_855_1_RIGID : Subsystem
  Part_923_1_RIGID : Subsystem
  Part_924_1_RIGID : Subsystem
  Part_925_1_RIGID : Subsystem
  ReferenceFrame : sm_lib/Frames and Transforms/Reference Frame
  Screw_10_3_4_in_1_RIGID : Subsystem
  Screw_10_3_4_in_2_RIGID : Subsystem
  Screw_10_3_4_in_3_RIGID : Subsystem
  Screw_10_3_4_in_4_RIGID : Subsystem
  Screw_8_1_2_in_1_RIGID : Subsystem
  Screw_8_1_2_in_2_RIGID : Subsystem
  Set_Screw_4_1_4_in_1_RIGID : Subsystem
  Set_Screw_4_1_4_in_2_RIGID : Subsystem
  Set_Screw_4_1_4_in_3_RIGID : Subsystem
  Set_Screw_4_1_4_in_4_RIGID : Subsystem
  Set_Screw_4_1_4_in_5_RIGID : Subsystem
  Set_Screw_4_1_4_in_6_RIGID : Subsystem
  Spacer_1_RIGID : Subsystem
  Spacer_2_RIGID : Subsystem
  Spacer_3_RIGID : Subsystem
  Spring_Pin_1_8_in_OD_1_4_in_L_10_RIGID : Subsystem
  Spring_Pin_1_8_in_OD_1_4_in_L_11_RIGID : Subsystem
  Spring_Pin_1_8_in_OD_1_4_in_L_12_RIGID : Subsystem
  Spring_Pin_1_8_in_OD_1_4_in_L_13_RIGID : Subsystem
  Spring_Pin_1_8_in_OD_1_4_in_L_14_RIGID : Subsystem
  Spring_Pin_1_8_in_OD_1_4_in_L_15_RIGID : Subsystem
  Spring_Pin_1_8_in_OD_1_4_in_L_16_RIGID : Subsystem
  Spring_Pin_1_8_in_OD_1_4_in_L_17_RIGID : Subsystem
  Spring_Pin_1_8_in_OD_1_4_in_L_18_RIGID : Subsystem
  Spring_Pin_1_8_in_OD_1_4_in_L_19_RIGID : Subsystem
  Spring_Pin_1_8_in_OD_1_4_in_L_1_RIGID : Subsystem
  Spring_Pin_1_8_in_OD_1_4_in_L_20_RIGID : Subsystem
  Spring_Pin_1_8_in_OD_1_4_in_L_21_RIGID : Subsystem
  Spring_Pin_1_8_in_OD_1_4_in_L_22_RIGID : Subsystem
  Spring_Pin_1_8_in_OD_1_4_in_L_2_RIGID : Subsystem
  Spring_Pin_1_8_in_OD_1_4_in_L_3_RIGID : Subsystem
  Spring_Pin_1_8_in_OD_1_4_in_L_4_RIGID : Subsystem
  Spring_Pin_1_8_in_OD_1_4_in_L_5_RIGID : Subsystem
  Spring_Pin_1_8_in_OD_1_4_in_L_6_RIGID : Subsystem
  Spring_Pin_1_8_in_OD_1_4_in_L_7_RIGID : Subsystem
  Spring_Pin_1_8_in_OD_1_4_in_L_8_RIGID : Subsystem
  Spring_Pin_1_8_in_OD_1_4_in_L_9_RIGID : Subsystem
  Standoff_1_RIGID : Subsystem
  Transform : sm_lib/Frames and Transforms/Rigid Transform  TranslationMethod=Cartesian  TranslationStandardOffset=0  TranslationLengthUnit=in  TranslationStandardAxis=+Z  TranslationCartesianOffset=frontParams.RigidTransform(422).translation  TranslationROffset=0  TranslationROffsetUnits=m  TranslationZOffset=0  TranslationZOffsetUnits=m  TranslationThetaOffset=0  TranslationThetaOffsetUnits=deg  RotationMethod=ArbitraryAxis  RotationAngleUnits=rad  RotationStandardAxis=+Z  RotationAngle=frontParams.RigidTransform(422).angle  RotationArbitraryAxis=frontParams.RigidTransform(422).axis  FollAlignAxisA=+X  BaseAlignAxisA=+Y  FollAlignAxisB=+Y  BaseAlignAxisB=+Z  RotationSequenceAxes=FollowerAxes  RotationSequence=XYX  RotationSequenceAngles=[0 0 0]  RotationSequenceAnglesUnits=deg  RotationMatrix=[1 0 0; 0 1 0; 0 0 1]
  Washer_10_1_RIGID : Subsystem
  Washer_10_2_RIGID : Subsystem
  Washer_10_3_RIGID : Subsystem
  Washer_10_4_RIGID : Subsystem
  Washer_8_1_RIGID : Subsystem
  Washer_8_2_RIGID : Subsystem
  bulkheads5_1_RIGID : Subsystem
  bulkheads5_2_RIGID : Subsystem
  bulkheads5_3_RIGID : Subsystem
  bulkheads5_4_RIGID : Subsystem
  bulkheads5_5_RIGID : Subsystem
  bulkheads6_1_RIGID : Subsystem
  bulkheads6_2_RIGID : Subsystem
  bulkheads6_3_RIGID : Subsystem
  bulkheads6_4_RIGID : Subsystem
  bulkheads6_5_RIGID : Subsystem
  forward_torso_l_1_RIGID : Subsystem
  forward_torso_r_1_RIGID : Subsystem
  F : PMIOPort  Side=Left
  F2 : PMIOPort  Port=2  Side=Left
  F1 : PMIOPort  Port=3  Side=Right
  connections:
  Bracket_2_RIGID/LConn1 -- Bracket_1_RIGID/LConn1 -- Bracket_3_RIGID/LConn1 -- Bracket_4_RIGID/LConn1 -- Bracket_5_RIGID/LConn1 -- Bracket_6_RIGID/LConn1 -- Hinge_1_RIGID/LConn1 -- Hinge_2_RIGID/LConn1 -- Hinge_3_RIGID/LConn1 -- Part_853_1_RIGID/LConn1 -- Part_854_1_RIGID/LConn1 -- Part_855_1_RIGID/LConn1 -- Part_923_1_RIGID/LConn1 -- Part_924_1_RIGID/LConn1 -- Part_925_1_RIGID/LConn1 -- Screw_10_3_4_in_1_RIGID/LConn1 -- Screw_10_3_4_in_2_RIGID/LConn1 -- Screw_10_3_4_in_3_RIGID/LConn1 -- Screw_10_3_4_in_4_RIGID/LConn1 -- Screw_8_1_2_in_1_RIGID/LConn1 -- Screw_8_1_2_in_2_RIGID/LConn1 -- Set_Screw_4_1_4_in_1_RIGID/LConn1 -- Set_Screw_4_1_4_in_2_RIGID/LConn1 -- Set_Screw_4_1_4_in_3_RIGID/LConn1 -- Set_Screw_4_1_4_in_4_RIGID/LConn1 -- Set_Screw_4_1_4_in_5_RIGID/LConn1 -- Set_Screw_4_1_4_in_6_RIGID/LConn1 -- Spacer_1_RIGID/LConn1 -- Spacer_2_RIGID/LConn1 -- Spacer_3_RIGID/LConn1 -- Spring_Pin_1_8_in_OD_1_4_in_L_10_RIGID/LConn1 -- Spring_Pin_1_8_in_OD_1_4_in_L_11_RIGID/LConn1 -- Spring_Pin_1_8_in_OD_1_4_in_L_12_RIGID/LConn1 -- Spring_Pin_1_8_in_OD_1_4_in_L_13_RIGID/LConn1 -- Spring_Pin_1_8_in_OD_1_4_in_L_14_RIGID/LConn1 -- Spring_Pin_1_8_in_OD_1_4_in_L_15_RIGID/LConn1 -- Spring_Pin_1_8_in_OD_1_4_in_L_16_RIGID/LConn1 -- Spring_Pin_1_8_in_OD_1_4_in_L_17_RIGID/LConn1 -- Spring_Pin_1_8_in_OD_1_4_in_L_18_RIGID/LConn1 -- Spring_Pin_1_8_in_OD_1_4_in_L_19_RIGID/LConn1 -- Spring_Pin_1_8_in_OD_1_4_in_L_1_RIGID/LConn1 -- Spring_Pin_1_8_in_OD_1_4_in_L_20_RIGID/LConn1 -- Spring_Pin_1_8_in_OD_1_4_in_L_21_RIGID/LConn1 -- Spring_Pin_1_8_in_OD_1_4_in_L_22_RIGID/LConn1 -- Spring_Pin_1_8_in_OD_1_4_in_L_2_RIGID/LConn1 -- Spring_Pin_1_8_in_OD_1_4_in_L_3_RIGID/LConn1 -- Spring_Pin_1_8_in_OD_1_4_in_L_4_RIGID/LConn1 -- Spring_Pin_1_8_in_OD_1_4_in_L_5_RIGID/LConn1 -- Spring_Pin_1_8_in_OD_1_4_in_L_6_RIGID/LConn1 -- Spring_Pin_1_8_in_OD_1_4_in_L_7_RIGID/LConn1 -- Spring_Pin_1_8_in_OD_1_4_in_L_8_RIGID/LConn1 -- Spring_Pin_1_8_in_OD_1_4_in_L_9_RIGID/LConn1 -- Standoff_1_RIGID/LConn1 -- Washer_10_1_RIGID/LConn1 -- Washer_10_2_RIGID/LConn1 -- Washer_10_3_RIGID/LConn1 -- Washer_10_4_RIGID/LConn1 -- Washer_8_1_RIGID/LConn1 -- Washer_8_2_RIGID/LConn1 -- bulkheads5_1_RIGID/LConn1 -- bulkheads5_2_RIGID/LConn1 -- bulkheads5_3_RIGID/LConn1 -- bulkheads5_4_RIGID/LConn1 -- bulkheads5_5_RIGID/LConn1 -- bulkheads6_1_RIGID/LConn1 -- bulkheads6_2_RIGID/LConn1 -- bulkheads6_3_RIGID/LConn1 -- bulkheads6_4_RIGID/LConn1 -- bulkheads6_5_RIGID/LConn1 -- forward_torso_l_1_RIGID/LConn1 -- forward_torso_r_1_RIGID/LConn3
  forward_torso_r_1_RIGID/LConn2 -- F/RConn1
  Spacer_2_RIGID/LConn2 -- F1/RConn1
  Hinge_1_RIGID/LConn2 -- F2/RConn1
  Transform/RConn1 -- forward_torso_r_1_RIGID/LConn1
  ReferenceFrame/RConn1 -- Transform/LConn1
